simulink model "TCML_Ex"  (R2015a)
settings: Solver=ode4  StartTime=0.0  StopTime=tsim  FixedStep=MWS.TC.Ext.dt  RelTol=1e-3
libraries: lib_TCML x3
settings Model: Creator=jlkratz  LastModifiedBy=jlkratz

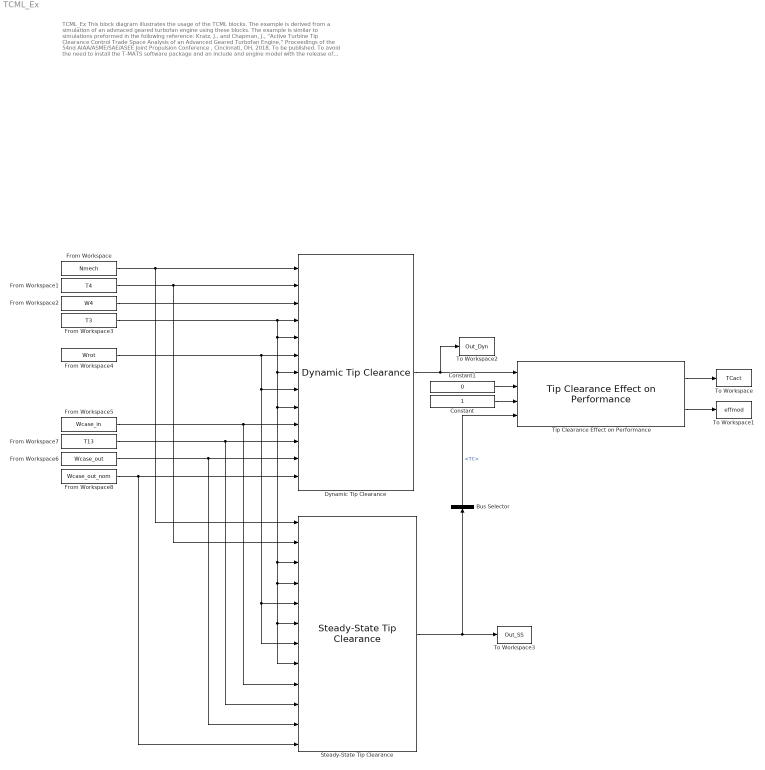
== system TCML_Ex ==
  note: TCML_Ex
      |
      | This block diagram illustrates the usage of the TCML blocks. The example is derived from a simulation of an advnaced geared turbofan engine using these
      | blocks. The example is similar to simulations preformed in the following reference:
      |
      | Kratz, J., and Chapman, J., “Active Turbine Tip Clearance Control Trade Space Analysis of an Advanced Geared Turbofan Engine,” Proceedings of the 54nd
      | AIAA/ASME/SAE/ASEE Joint Propulsion Conference , Cincinnati, OH, 2018. To be published.
      |
      | To avoid the need to install the T-MATS software package and an include and engine model with the release of TCML for the purpose of this example, the
      | tip clearance blocks are executed in an open-loop manner. The inputs are supplied by "from workspace" block which contain data extracted from a
      | simulation of the AGTF30 engine which is described in the following references.
      |
      | Jones, S.M., Haller, W.J., Tong, M.T., “An N+3 Technology Level Reference Propulsion System”, NASA/TM-2017-219501, 2017.
      | Chapman, J., and Litt, J., “Control Design for an Advanced Geared Turbofan Engine,” AIAA Propulsion and Energy Forum , Atlanta, GA, 2017.
      |
      | If an engine model were present in the simulation, the efficiency modifier would be an input into the engine simulation to modify the component efficency
      | and the inputs to the tip clearance model would be supplied directly from the engine simulation. if the tip clearance blocks were to be integrated with an
      | engine simulation, memory blocks may be necessary to prevent algebraic loops.
      |
      | Note: In this example, dynamic and steady state tip clearance blocks simulate the same configuration. Therefore, the tip clearance from the steady-state block
      | should match the nominal tip clearance from the dynamic tip clearance block. Therefore, the "NomConfig_M" option in the "Tip Clearance Effect on
      | Performance" block is not necessary but has been activated to illustrate its use in a more general case.
      |
      | The workspace for this example is initialized by the run_TCML_Ex.m file. Executing that file will also start the simulation of this model and produce several
      | plots to display the results.
  Bus Selector : BusSelector  OutputSignals=TC
  Constant : Constant
  Constant1 : Constant  Value=0
  Dynamic Tip Clearance : lib_TCML/Dynamic Tip Clearance  m_Blade_M=MWS.TC.Blade.m  A_Blade_M=MWS.TC.Blade.A  Cp_TempDependence_Blade_M=on  Cp_Blade_M=4.5  TCp_Blade_Data_M=MWS.TC.Blade.TCp_Data  Cp_Blade_Data_M=MWS.TC.Blade.Cp_Data  eta_Blade_M=MWS.TC.Blade.eta  T0_Blade_M=MWS.TC.Blade.T0  dt_Blade_M=MWS.TC.Blade.dt  h_Const_Blade_M=off  h_Eqn_Blade_M=on  h_Data_Blade_M=off  h_Blade_M=0.03  hcoeff_Blade_M=MWS.TC.Blade.hcoeff  Wdes_Blade_M=MWS.TC.Blade.Wdes  Tdes_Blade_M=MWS.TC.Blade.Tdes  Wc_Blade_Data_M=[0 100]  Tc_Blade_Data_M=[0 10]  h_Blade_Data_M=[0.03 0.03; 0.03 0.03]  L_Blade_M=MWS.TC.Blade.L0  rho_Blade_M=MWS.TC.Blade.rho  alpha_TempDependence_Blade_M=on  alpha_Blade_M=0.000008  Talpha_Blade_Data_M=MWS.TC.Blade.Talpha_Data  alpha_Blade_Data_M=MWS.TC.Blade.alpha_Data  E_TempDependence_Blade_M=on  E_Blade_M=3974400000  TE_Blade_Data_M=MWS.TC.Blade.TE_Data  E_Blade_Data_M=MWS.TC.Blade.E_Data  W_Rotor_M=MWS.TC.Rotor.W  n_Rotor_M=MWS.TC.Rotor.n  T0_Rotor_M=MWS.TC.Rotor.T0  dt_Rotor_M=MWS.TC.Rotor.dt  rho_Rotor_M=MWS.TC.Rotor.rho  k_TempDependence_Rotor_M=on  k_Rotor_M=0.0015  Tk_Rotor_Data_M=MWS.TC.Rotor.Tk_Data  k_Rotor_Data_M=MWS.TC.Rotor.k_Data  Cp_TempDependence_Rotor_M=on  Cp_Rotor_M=4.5  TCp_Rotor_Data_M=MWS.TC.Rotor.TCp_Data  Cp_Rotor_Data_M=MWS.TC.Rotor.Cp_Data  h_Const_Rotor_Front_M=off  h_Eqn_Rotor_Front_M=on  h_Data_Rotor_Front_M=off  h_Rotor_Front_M=0.03  hcoeff_Rotor_Front_M=MWS.TC.Rotor.hcoeff_front  Wdes_Rotor_Front_M=MWS.TC.Rotor.Wdes_front  Tdes_Rotor_Front_M=MWS.TC.Rotor.Tdes_front  Wc_Rotor_Front_Data_M=[0 100]  Tc_Rotor_Front_Data_M=[0 10]  h_Rotor_Front_Data_M=[0.003 0.003; 0.003 0.003]  h_Const_Rotor_Back_M=off  h_Eqn_Rotor_Back_M=on  h_Data_Rotor_Back_M=off  h_Rotor_Back_M=0.03  hcoeff_Rotor_Back_M=MWS.TC.Rotor.hcoeff_back  Wdes_Rotor_Back_M=MWS.TC.Rotor.Wdes_back  Tdes_Rotor_Back_M=MWS.TC.Rotor.Tdes_back  Wc_Rotor_Back_Data_M=[0 100]  Tc_Rotor_Back_Data_M=[0 10]  h_Rotor_Back_Data_M=[0.003 0.003; 0.003 0.003]  Ro_Rotor_M=MWS.TC.Rotor.Ro  alpha_TempDependence_Rotor_M=on  alpha_Rotor_M=0.000008  Talpha_Rotor_Data_M=MWS.TC.Rotor.Talpha_Data  alpha_Rotor_Data_M=MWS.TC.Rotor.alpha_Data  E_TempDependence_Rotor_M=on  E_Rotor_M=3974400000  TE_Rotor_Data_M=MWS.TC.Rotor.TE_Data  E_Rotor_Data_M=MWS.TC.Rotor.E_Data  v_TempDependence_Rotor_M=on  v_Rotor_M=0.3  Tv_Rotor_Data_M=MWS.TC.Rotor.Tv_Data  v_Rotor_Data_M=MWS.TC.Rotor.v_Data  W_Case_M=MWS.TC.Case.W  n_Case_M=MWS.TC.Case.n  T0_Case_M=MWS.TC.Case.T0  dt_Case_M=MWS.TC.Case.dt  rho_Case_M=MWS.TC.Case.rho  k_TempDependence_Case_M=on  k_Case_M=0.0015  Tk_Case_Data_M=MWS.TC.Case.Tk_Data  k_Case_Data_M=MWS.TC.Case.k_Data  Cp_TempDependence_Case_M=on  Cp_Case_M=4.5  TCp_Case_Data_M=MWS.TC.Case.TCp_Data  Cp_Case_Data_M=MWS.TC.Case.Cp_Data  h_Const_Case_In_M=off  h_Eqn_Case_In_M=on  h_Data_Case_In_M=off  h_Case_In_M=0.004  hcoeff_Case_In_M=MWS.TC.Case.hcoeff_in  Wdes_Case_In_M=MWS.TC.Case.Wdes_in  Tdes_Case_In_M=MWS.TC.Case.Tdes_in  Wc_Case_In_Data_M=[0 100]  Tc_Case_In_Data_M=[0 10]  h_Case_In_Data_M=[0.004 0.004; 0.004 0.004]  h_Const_Case_Out_M=off  h_Eqn_Case_Out_M=on  h_Data_Case_Out_M=off  h_Case_Out_M=0.004  hcoeff_Case_Out_M=MWS.TC.Case.hcoeff_out  Wdes_Case_Out_M=MWS.TC.Case.Wdes_out  Tdes_Case_Out_M=MWS.TC.Case.Tdes_out  Wc_Case_Out_Data_M=[0 100]  Tc_Case_Out_Data_M=[0 10]  h_Case_Out_Data_M=[0.003 0.003; 0.003 0.003]  Ri_Case_M=MWS.TC.Case.Ri  L_Shroud_M=MWS.TC.L_Shroud  alpha_TempDependence_Case_M=on  alpha_Case_M=0.000008  Talpha_Case_Data_M=MWS.TC.Case.Talpha_Data  alpha_Case_Data_M=MWS.TC.Case.alpha_Data  dt_M=MWS.TC.Ext.dt  T0_Core_M=MWS.TC.FC.T0_Core  W0_Core_M=MWS.TC.FC.W0_Core  Tcool0_Blade_M=MWS.TC.FC.Tcool0_Blade  Tcool0_Rotor_Front_M=MWS.TC.FC.Tcool0_Rotor_Front  Wcool0_Rotor_Front_M=MWS.TC.FC.Wcool0_Rotor_Front  Tcool0_Rotor_Back_M=MWS.TC.FC.Tcool0_Rotor_Back  Wcool0_Rotor_Back_M=MWS.TC.FC.Wcool0_Rotor_Back  Tcool0_Case_In_M=MWS.TC.FC.Tcool0_Case_In  Wcool0_Case_In_M=MWS.TC.FC.Wcool0_Case_In  Tcool0_Case_Out_M=MWS.TC.FC.Tcool0_Case_Out  Wcool0_Case_Out_M=MWS.TC.FC.Wcool0_Case_Out  Wcool0_Case_Out_Nom_M=MWS.TC.FC.Wcool0_Case_Out_Nom
  From Workspace : FromWorkspace  VariableName=Nmech  SampleTime=0
  From Workspace1 : FromWorkspace  VariableName=T4  SampleTime=0
  From Workspace2 : FromWorkspace  VariableName=W4  SampleTime=0
  From Workspace3 : FromWorkspace  VariableName=T3  SampleTime=0
  From Workspace4 : FromWorkspace  VariableName=Wrot  SampleTime=0
  From Workspace5 : FromWorkspace  VariableName=Wcase_in  SampleTime=0
  From Workspace6 : FromWorkspace  VariableName=Wcase_out  SampleTime=0
  From Workspace7 : FromWorkspace  VariableName=T13  SampleTime=0
  From Workspace8 : FromWorkspace  VariableName=Wcase_out_nom  SampleTime=0
  Steady-State Tip Clearance : lib_TCML/Steady-State Tip Clearance  eta_Blade_M=MWS.TC.Blade.eta  T0_Blade_M=MWS.TC.Blade.T0  h_Const_Blade_M=off  h_Eqn_Blade_M=on  h_Data_Blade_M=off  h_Blade_M=0.03  hcoeff_Blade_M=MWS.TC.Blade.hcoeff  Wdes_Blade_M=MWS.TC.Blade.Wdes  Tdes_Blade_M=MWS.TC.Blade.Tdes  Wc_Blade_Data_M=[0 100]  Tc_Blade_Data_M=[0 10]  h_Blade_Data_M=[0.03 0.03; 0.03 0.03]  L_Blade_M=MWS.TC.Blade.L0  rho_Blade_M=MWS.TC.Blade.rho  alpha_TempDependence_Blade_M=on  alpha_Blade_M=0.000008  Talpha_Blade_Data_M=MWS.TC.Blade.Talpha_Data  alpha_Blade_Data_M=MWS.TC.Blade.alpha_Data  E_TempDependence_Blade_M=on  E_Blade_M=3974400000  TE_Blade_Data_M=MWS.TC.Blade.TE_Data  E_Blade_Data_M=MWS.TC.Blade.E_Data  W_Rotor_M=MWS.TC.Rotor.W  n_Rotor_M=MWS.TC.Rotor.n  T0_Rotor_M=MWS.TC.Rotor.T0  rho_Rotor_M=MWS.TC.Rotor.rho  k_TempDependence_Rotor_M=on  k_Rotor_M=0.0015  Tk_Rotor_Data_M=MWS.TC.Rotor.Tk_Data  k_Rotor_Data_M=MWS.TC.Rotor.k_Data  h_Const_Rotor_Front_M=off  h_Eqn_Rotor_Front_M=on  h_Data_Rotor_Front_M=off  h_Rotor_Front_M=0.03  hcoeff_Rotor_Front_M=MWS.TC.Rotor.hcoeff_front  Wdes_Rotor_Front_M=MWS.TC.Rotor.Wdes_front  Tdes_Rotor_Front_M=MWS.TC.Rotor.Tdes_front  Wc_Rotor_Front_Data_M=[0 100]  Tc_Rotor_Front_Data_M=[0 10]  h_Rotor_Front_Data_M=[0.003 0.003; 0.003 0.003]  h_Const_Rotor_Back_M=off  h_Eqn_Rotor_Back_M=on  h_Data_Rotor_Back_M=off  h_Rotor_Back_M=0.03  hcoeff_Rotor_Back_M=MWS.TC.Rotor.hcoeff_back  Wdes_Rotor_Back_M=MWS.TC.Rotor.Wdes_back  Tdes_Rotor_Back_M=MWS.TC.Rotor.Tdes_back  Wc_Rotor_Back_Data_M=[0 100]  Tc_Rotor_Back_Data_M=[0 10]  h_Rotor_Back_Data_M=[0.003 0.003; 0.003 0.003]  Ro_Rotor_M=MWS.TC.Rotor.Ro  alpha_TempDependence_Rotor_M=on  alpha_Rotor_M=0.000008  Talpha_Rotor_Data_M=MWS.TC.Rotor.Talpha_Data  alpha_Rotor_Data_M=MWS.TC.Rotor.alpha_Data  E_TempDependence_Rotor_M=on  E_Rotor_M=3974400000  TE_Rotor_Data_M=MWS.TC.Rotor.TE_Data  E_Rotor_Data_M=MWS.TC.Rotor.E_Data  v_TempDependence_Rotor_M=on  v_Rotor_M=0.3  Tv_Rotor_Data_M=MWS.TC.Rotor.Tv_Data  v_Rotor_Data_M=MWS.TC.Rotor.v_Data  W_Case_M=MWS.TC.Case.W  n_Case_M=MWS.TC.Case.n  T0_Case_M=MWS.TC.Case.T0  rho_Case_M=MWS.TC.Case.rho  k_TempDependence_Case_M=on  k_Case_M=0.0015  Tk_Case_Data_M=MWS.TC.Case.Tk_Data  k_Case_Data_M=MWS.TC.Case.k_Data  h_Const_Case_In_M=off  h_Eqn_Case_In_M=on  h_Data_Case_In_M=off  h_Case_In_M=0.02  hcoeff_Case_In_M=MWS.TC.Case.hcoeff_in  Wdes_Case_In_M=MWS.TC.Case.Wdes_in  Tdes_Case_In_M=MWS.TC.Case.Tdes_in  Wc_Case_In_Data_M=[0 100]  Tc_Case_In_Data_M=[1 10]  h_Case_In_Data_M=[0.02 0.02; 0.02 0.02]  h_Const_Case_Out_M=off  h_Eqn_Case_Out_M=on  h_Data_Case_Out_M=off  h_Case_Out_M=0.01  hcoeff_Case_Out_M=MWS.TC.Case.hcoeff_out  Wdes_Case_Out_M=MWS.TC.Case.Wdes_out  Tdes_Case_Out_M=MWS.TC.Case.Tdes_out  Wc_Case_Out_Data_M=[0 100]  Tc_Case_Out_Data_M=[0 10]  h_Case_Out_Data_M=[0.01 0.01; 0.01 0.01]  Ri_Case_M=MWS.TC.Case.Ri  L_Shroud_M=MWS.TC.L_Shroud  alpha_TempDependence_Case_M=on  alpha_Case_M=0.000008  Talpha_Case_Data_M=MWS.TC.Case.Talpha_Data  alpha_Case_Data_M=MWS.TC.Case.alpha_Data
  Tip Clearance Effect on Performance : lib_TCML/Tip Clearance Effect on Performance  L_Shroud_M=MWS.TC.L_Shroud  DegGap_M=MWS.TC.DegGap  NomConfig_M=on
  To Workspace : ToWorkspace  VariableName=TCact  SaveFormat=Timeseries  SampleTime=-1
  To Workspace1 : ToWorkspace  VariableName=effmod  SaveFormat=Timeseries  SampleTime=-1
  To Workspace2 : ToWorkspace  VariableName=Out_Dyn  SaveFormat=Timeseries  SampleTime=-1
  To Workspace3 : ToWorkspace  VariableName=Out_SS  SaveFormat=Timeseries  SampleTime=-1
  wires:
  Steady-State Tip Clearance/1 -> To Workspace3/1, Bus Selector/1
  Constant/1 -> Tip Clearance Effect on Performance/3
  Constant1/1 -> Tip Clearance Effect on Performance/2
  Dynamic Tip Clearance/1 -> To Workspace2/1, Tip Clearance Effect on Performance/1
  Tip Clearance Effect on Performance/1 -> To Workspace/1
  Tip Clearance Effect on Performance/2 -> To Workspace1/1
  From Workspace/1 -> Steady-State Tip Clearance/1, Dynamic Tip Clearance/1
  From Workspace1/1 -> Steady-State Tip Clearance/2, Dynamic Tip Clearance/2
  From Workspace2/1 -> Dynamic Tip Clearance/3
  From Workspace3/1 -> Steady-State Tip Clearance/8, Steady-State Tip Clearance/6, Steady-State Tip Clearance/4, Steady-State Tip Clearance/3, Dynamic Tip Clearance/9, Dynamic Tip Clearance/7, Dynamic Tip Clearance/5, Dynamic Tip Clearance/4
  From Workspace4/1 -> Steady-State Tip Clearance/7, Steady-State Tip Clearance/5, Dynamic Tip Clearance/8, Dynamic Tip Clearance/6
  From Workspace5/1 -> Steady-State Tip Clearance/9, Dynamic Tip Clearance/10
  From Workspace7/1 -> Steady-State Tip Clearance/10, Dynamic Tip Clearance/11
  From Workspace8/1 -> Steady-State Tip Clearance/12, Dynamic Tip Clearance/13
  Bus Selector/1 -> Tip Clearance Effect on Performance/4  "<TC>"
  From Workspace6/1 -> Steady-State Tip Clearance/11, Dynamic Tip Clearance/12
